simulink model "HW_9"  (Simulink 7.9)
settings: Solver=ode45  StartTime=0.0  StopTime=10.0  RelTol=1e-3
settings Model: Creator=alex  LastModifiedBy=alex

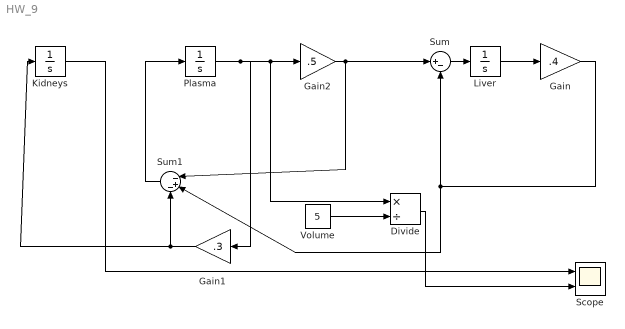
== system HW_9 ==
  Divide : Product  Inputs=*/
  Gain : Gain  Gain=.4
  Gain1 : Gain  Gain=.3
  Gain2 : Gain  Gain=.5
  Kidneys : Integrator
  Liver : Integrator
  Plasma : Integrator  InitialCondition=200
  Scope : Scope  NumInputPorts=2
      settings: YMin=-5~-5  YMax=5~5
  Sum : Sum  Inputs=|+-
  Sum1 : Sum  Inputs=|-+-
  Volume : Constant  Value=5
  wires:
  Plasma/1 -> Gain1/1, Gain2/1, Divide/1
  Gain2/1 -> Sum1/1, Sum/1
  Sum1/1 -> Plasma/1
  Sum/1 -> Liver/1
  Liver/1 -> Gain/1
  Gain/1 -> Sum/2, Sum1/2
  Gain1/1 -> Sum1/3, Kidneys/1
  Kidneys/1 -> Scope/1
  Volume/1 -> Divide/2
  Divide/1 -> Scope/2
